simulink model "EV_Model"  (R2020b)
settings: Solver=VariableStepAuto  StartTime=0.0  StopTime=inf  RelTol=1e-3
undefined symbols (not defined in the file): battery, DCDC, DCU, DCU1, DiscIntNeverNeededParam, ECP, HVH, magnitude, PAR, PTC, road, SampleTime, VCU, veh, wheel
libraries: simulink x10
(part 1 of 2)
settings Model: SimulationMode=accelerator  Creator=LIKAI  LastModifiedBy=LIKAI

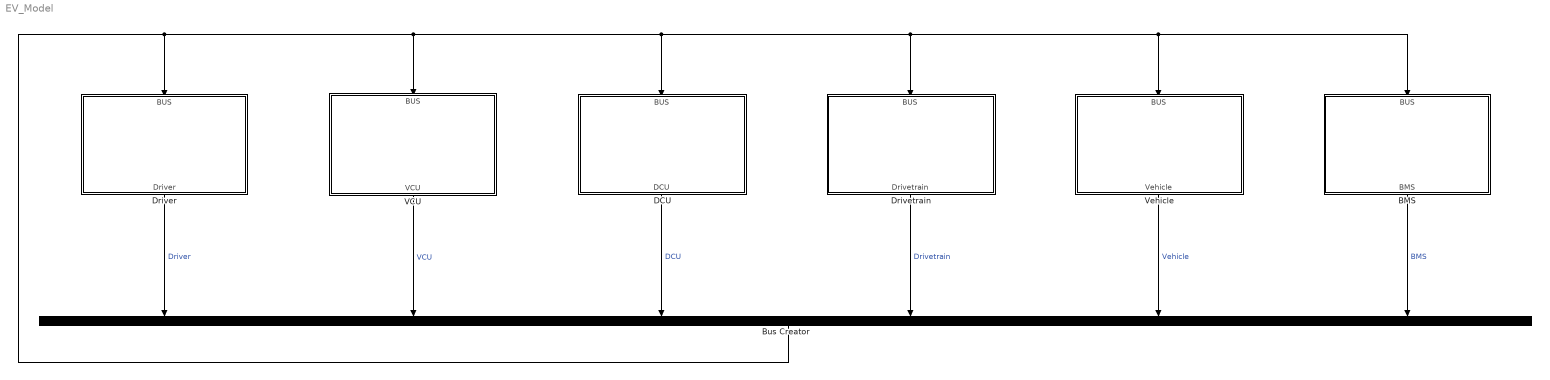
== system EV_Model ==
  BMS : Subsystem
      settings: PortSchema="{\"entries\":[{\"content\":{\"sides\":[{\"content\":{\"connectorIds\":[]},\"type\":\"ConnectorPlacement.EquallySpacedRectSide\",\"uuid\":\"ede90b11-bc22-42fb-ada4-d3cc8cd7e01b\"},{\"content\":{\"connectorIds\":[],\"side\":\"RIGHT\"},\"type\":\"ConnectorPlacement.EquallySpacedRectSide\",\"uuid\":\"291a790d-3ed9-499e-8b51-4c4b7bb0ca71\"},{\"content\":{\"connectorIds\":[\"In1\"],\"side\":\"TOP\"},\"type\":\"ConnectorPlacement.EquallySpacedRectSide\",\"uuid\":\"427db5b2-2806-4b1c-ab96-e85c737f1799\"},{\"content\":{\"connectorIds\":[\"Out1\"],\"side\":\"BOTTOM\"},\"type\":\"ConnectorPlacement.EquallySpacedRectSide\",\"uuid\":\"1165d243-ed6a-4f50-80fe-e5443602b1fc\"},{\"content\":{\"connectorIds\":[],\"side\":\"HIDDEN\"},\"type\":\"ConnectorPlacement.EquallySpacedRectSide\",\"uuid\":\"de95d8f7-8967-4dbd-bf20-0c2997ce61ce\"}]},\"type\":\"ConnectorPlacement.EquallySpacedConnector\",\"uuid\":\"60485ffc-06b9-4405-b269-3de14a5dc818\"}],\"packageUris\":[\"http://schema.mathworks.com/mf0/Connector/R2020b\"],\"version\":\"1.0\"}"
  Bus Creator : BusCreator  Inputs=6
  DCU : Subsystem
      settings: PortSchema="{\"entries\":[{\"content\":{\"sides\":[{\"content\":{\"connectorIds\":[]},\"type\":\"ConnectorPlacement.EquallySpacedRectSide\",\"uuid\":\"ede90b11-bc22-42fb-ada4-d3cc8cd7e01b\"},{\"content\":{\"connectorIds\":[],\"side\":\"RIGHT\"},\"type\":\"ConnectorPlacement.EquallySpacedRectSide\",\"uuid\":\"291a790d-3ed9-499e-8b51-4c4b7bb0ca71\"},{\"content\":{\"connectorIds\":[\"In1\"],\"side\":\"TOP\"},\"type\":\"ConnectorPlacement.EquallySpacedRectSide\",\"uuid\":\"427db5b2-2806-4b1c-ab96-e85c737f1799\"},{\"content\":{\"connectorIds\":[\"Out1\"],\"side\":\"BOTTOM\"},\"type\":\"ConnectorPlacement.EquallySpacedRectSide\",\"uuid\":\"f52060db-3c77-45a1-a434-e300d9b83897\"},{\"content\":{\"connectorIds\":[],\"side\":\"HIDDEN\"},\"type\":\"ConnectorPlacement.EquallySpacedRectSide\",\"uuid\":\"de95d8f7-8967-4dbd-bf20-0c2997ce61ce\"}]},\"type\":\"ConnectorPlacement.EquallySpacedConnector\",\"uuid\":\"60485ffc-06b9-4405-b269-3de14a5dc818\"}],\"packageUris\":[\"http://schema.mathworks.com/mf0/Connector/R2020b\"],\"version\":\"1.0\"}"
  Driver : Subsystem
      settings: PortSchema="{\"entries\":[{\"content\":{\"sides\":[{\"content\":{\"connectorIds\":[]},\"type\":\"ConnectorPlacement.EquallySpacedRectSide\",\"uuid\":\"ede90b11-bc22-42fb-ada4-d3cc8cd7e01b\"},{\"content\":{\"connectorIds\":[],\"side\":\"RIGHT\"},\"type\":\"ConnectorPlacement.EquallySpacedRectSide\",\"uuid\":\"291a790d-3ed9-499e-8b51-4c4b7bb0ca71\"},{\"content\":{\"connectorIds\":[\"In1\"],\"side\":\"TOP\"},\"type\":\"ConnectorPlacement.EquallySpacedRectSide\",\"uuid\":\"427db5b2-2806-4b1c-ab96-e85c737f1799\"},{\"content\":{\"connectorIds\":[\"Out1\"],\"side\":\"BOTTOM\"},\"type\":\"ConnectorPlacement.EquallySpacedRectSide\",\"uuid\":\"a05f4215-27ad-4dfe-901f-55fb3061c621\"},{\"content\":{\"connectorIds\":[],\"side\":\"HIDDEN\"},\"type\":\"ConnectorPlacement.EquallySpacedRectSide\",\"uuid\":\"de95d8f7-8967-4dbd-bf20-0c2997ce61ce\"}]},\"type\":\"ConnectorPlacement.EquallySpacedConnector\",\"uuid\":\"60485ffc-06b9-4405-b269-3de14a5dc818\"}],\"packageUris\":[\"http://schema.mathworks.com/mf0/Connector/R2020b\"],\"version\":\"1.0\"}"
  Drivetrain : Subsystem
      settings: PortSchema="{\"entries\":[{\"content\":{\"sides\":[{\"content\":{\"connectorIds\":[]},\"type\":\"ConnectorPlacement.EquallySpacedRectSide\",\"uuid\":\"ede90b11-bc22-42fb-ada4-d3cc8cd7e01b\"},{\"content\":{\"connectorIds\":[],\"side\":\"RIGHT\"},\"type\":\"ConnectorPlacement.EquallySpacedRectSide\",\"uuid\":\"291a790d-3ed9-499e-8b51-4c4b7bb0ca71\"},{\"content\":{\"connectorIds\":[\"In1\"],\"side\":\"TOP\"},\"type\":\"ConnectorPlacement.EquallySpacedRectSide\",\"uuid\":\"427db5b2-2806-4b1c-ab96-e85c737f1799\"},{\"content\":{\"connectorIds\":[\"Out1\"],\"side\":\"BOTTOM\"},\"type\":\"ConnectorPlacement.EquallySpacedRectSide\",\"uuid\":\"40f490df-ef26-4730-ad02-e07a11bb8b70\"},{\"content\":{\"connectorIds\":[],\"side\":\"HIDDEN\"},\"type\":\"ConnectorPlacement.EquallySpacedRectSide\",\"uuid\":\"de95d8f7-8967-4dbd-bf20-0c2997ce61ce\"}]},\"type\":\"ConnectorPlacement.EquallySpacedConnector\",\"uuid\":\"60485ffc-06b9-4405-b269-3de14a5dc818\"}],\"packageUris\":[\"http://schema.mathworks.com/mf0/Connector/R2020b\"],\"version\":\"1.0\"}"
  VCU : Subsystem
      settings: PortSchema="{\"entries\":[{\"content\":{\"sides\":[{\"content\":{\"connectorIds\":[]},\"type\":\"ConnectorPlacement.EquallySpacedRectSide\",\"uuid\":\"ede90b11-bc22-42fb-ada4-d3cc8cd7e01b\"},{\"content\":{\"connectorIds\":[],\"side\":\"RIGHT\"},\"type\":\"ConnectorPlacement.EquallySpacedRectSide\",\"uuid\":\"291a790d-3ed9-499e-8b51-4c4b7bb0ca71\"},{\"content\":{\"connectorIds\":[\"In1\"],\"side\":\"TOP\"},\"type\":\"ConnectorPlacement.EquallySpacedRectSide\",\"uuid\":\"427db5b2-2806-4b1c-ab96-e85c737f1799\"},{\"content\":{\"connectorIds\":[\"Out1\"],\"side\":\"BOTTOM\"},\"type\":\"ConnectorPlacement.EquallySpacedRectSide\",\"uuid\":\"15192dcd-7739-45f8-9f11-3c35b4b9a8fd\"},{\"content\":{\"connectorIds\":[],\"side\":\"HIDDEN\"},\"type\":\"ConnectorPlacement.EquallySpacedRectSide\",\"uuid\":\"de95d8f7-8967-4dbd-bf20-0c2997ce61ce\"}]},\"type\":\"ConnectorPlacement.EquallySpacedConnector\",\"uuid\":\"60485ffc-06b9-4405-b269-3de14a5dc818\"}],\"packageUris\":[\"http://schema.mathworks.com/mf0/Connector/R2020b\"],\"version\":\"1.0\"}"
  Vehicle : Subsystem
      settings: PortSchema="{\"entries\":[{\"content\":{\"sides\":[{\"content\":{\"connectorIds\":[]},\"type\":\"ConnectorPlacement.EquallySpacedRectSide\",\"uuid\":\"ede90b11-bc22-42fb-ada4-d3cc8cd7e01b\"},{\"content\":{\"connectorIds\":[],\"side\":\"RIGHT\"},\"type\":\"ConnectorPlacement.EquallySpacedRectSide\",\"uuid\":\"291a790d-3ed9-499e-8b51-4c4b7bb0ca71\"},{\"content\":{\"connectorIds\":[\"In1\"],\"side\":\"TOP\"},\"type\":\"ConnectorPlacement.EquallySpacedRectSide\",\"uuid\":\"427db5b2-2806-4b1c-ab96-e85c737f1799\"},{\"content\":{\"connectorIds\":[\"Out1\"],\"side\":\"BOTTOM\"},\"type\":\"ConnectorPlacement.EquallySpacedRectSide\",\"uuid\":\"01d5a7f7-95dc-4d6a-a6a5-fe54827ab0e5\"},{\"content\":{\"connectorIds\":[],\"side\":\"HIDDEN\"},\"type\":\"ConnectorPlacement.EquallySpacedRectSide\",\"uuid\":\"de95d8f7-8967-4dbd-bf20-0c2997ce61ce\"}]},\"type\":\"ConnectorPlacement.EquallySpacedConnector\",\"uuid\":\"60485ffc-06b9-4405-b269-3de14a5dc818\"}],\"packageUris\":[\"http://schema.mathworks.com/mf0/Connector/R2020b\"],\"version\":\"1.0\"}"
  wires:
  VCU/1(VCU) -> Bus Creator/2  "VCU"
  Driver/1(Driver) -> Bus Creator/1  "Driver"
  DCU/1(DCU) -> Bus Creator/3  "DCU"
  Drivetrain/1(Drivetrain) -> Bus Creator/4  "Drivetrain"
  Vehicle/1(Vehicle) -> Bus Creator/5  "Vehicle"
  BMS/1(BMS) -> Bus Creator/6  "BMS"
  Bus Creator/1 -> Drivetrain/1(BUS), BMS/1(BUS), Vehicle/1(BUS), DCU/1(BUS), VCU/1(BUS), Driver/1(BUS)

== system EV_Model/BMS ==
  BUS : Inport
  Battery Management System : Subsystem
  Bus Creator1 : BusCreator  Inputs=4
  Bus Selector : BusSelector  OutputSignals=Vehicle.AcesPwr_kW,Drivetrain.BattPwrReq_kW
  BMS : Outport  VectorParamsAs1DForOutWhenUnconnected=off
  wires:
  BUS/1 -> Bus Selector/1
  Battery Management System/1(BattSOC_1) -> Bus Creator1/1  "BattSOC_1"
  Battery Management System/2(BattVolt_V) -> Bus Creator1/2  "BattVolt_V"
  Battery Management System/3(BattPwrDischrgLmt_kW) -> Bus Creator1/3  "BattPwrDischrgLmt_kW"
  Battery Management System/4(BattPwrChrgLmt_kW) -> Bus Creator1/4  "BattPwrChrgLmt_kW"
  Bus Creator1/1 -> BMS/1
  Bus Selector/1 -> Battery Management System/1(AcesPwr_kW)  "<AcesPwr_kW>"
  Bus Selector/2 -> Battery Management System/2(BattPwrReq_kW)  "<BattPwrReq_kW>"

== system EV_Model/DCU ==
  BUS : Inport
  Bus Creator : BusCreator  Inputs=4
  Bus Selector : BusSelector  OutputSignals=BMS.BattVolt_V,Drivetrain.MotSpdAct_rpm,VCU.MotTrqReqBattPwrLimit_Nm
  Subsystem : Subsystem
  DCU : Outport  VectorParamsAs1DForOutWhenUnconnected=off
  wires:
  BUS/1 -> Bus Selector/1
  Bus Creator/1 -> DCU/1
  Subsystem/1(DCUTrqLimit_Nm) -> Bus Creator/1  "DCUTrqLimit_Nm"
  Subsystem/2(DCUPwrLimit_Nm) -> Bus Creator/2  "DCUPwrLimit_Nm"
  Subsystem/3(MotEffi2K_1) -> Bus Creator/3  "MotEffi2K_1"
  Subsystem/4(MotPwrElecReq_kW) -> Bus Creator/4  "MotPwrElecReq_kW"
  Bus Selector/1 -> Subsystem/1(BattVolt_V)  "<BattVolt_V>"
  Bus Selector/2 -> Subsystem/2(MotSpdAct_rpm)  "<MotSpdAct_rpm>"
  Bus Selector/3 -> Subsystem/3(MotTrqCmd_Nm)  "<MotTrqReqBattPwrLimit_Nm>"

== system EV_Model/Driver ==
  BUS : Inport
  Bus Creator : BusCreator  Inputs=2
  Bus Selector : BusSelector  OutputSignals=Vehicle.VehVelAct_kph
  DataTypeConversion1 : DataTypeConversion  OutDataTypeStr=double
  DataTypeConversion2 : DataTypeConversion  OutDataTypeStr=double
  DataTypeConversion6 : DataTypeConversion  OutDataTypeStr=double
  DriverModel : Subsystem
  Driver : Outport  VectorParamsAs1DForOutWhenUnconnected=off
  wires:
  Bus Selector/1 -> DataTypeConversion2/1  "<VehVelAct_kph>"
  DataTypeConversion2/1 -> DriverModel/1(VehVelAct_kph)
  DataTypeConversion1/1 -> Bus Creator/2  "WhlTrqCmd_Nm"
  DriverModel/1(VehVelTrgt_kph) -> DataTypeConversion6/1
  Bus Creator/1 -> Driver/1
  DriverModel/2(WhlTrqCmd_Nm) -> DataTypeConversion1/1
  BUS/1 -> Bus Selector/1
  DataTypeConversion6/1 -> Bus Creator/1  "VehVelTrgt_kph"

== system EV_Model/Drivetrain ==
  BUS : Inport
  Bus Creator : BusCreator  Inputs=4
  Bus Selector : BusSelector  OutputSignals=BMS.BattVolt_V,VCU.MotTrqFinalCmd_Nm,Vehicle.VehVelAct_kph
  Subsystem : Subsystem
  Drivetrain : Outport  VectorParamsAs1DForOutWhenUnconnected=off
  wires:
  Bus Creator/1 -> Drivetrain/1
  BUS/1 -> Bus Selector/1
  Subsystem/2(BattPwrReq_kW) -> Bus Creator/2  "BattPwrReq_kW"
  Subsystem/1(MotEffi_1) -> Bus Creator/1  "MotEffi_1"
  Subsystem/3(WheelTrqFromMot_Nm) -> Bus Creator/3  "WheelTrqFromMot_Nm"
  Subsystem/4(MotSpdAct_rpm) -> Bus Creator/4  "MotSpdAct_rpm"
  Bus Selector/3 -> Subsystem/3(VehVelAct_kph)  "<VehVelAct_kph>"
  Bus Selector/2 -> Subsystem/2(MotTrqCmd_Nm)  "<MotTrqFinalCmd_Nm>"
  Bus Selector/1 -> Subsystem/1(BattVolt_V)  "<BattVolt_V>"

== system EV_Model/VCU ==
  BUS : Inport
  Bus Creator : BusCreator  Inputs=2
  Bus Selector : BusSelector  OutputSignals=Driver.WhlTrqCmd_Nm,DCU.DCUTrqLimit_Nm,Vehicle.VehVelAct_kph,Drivetrain.MotSpdAct_rpm,DCU.MotPwrElecReq_kW,BMS.BattSOC_1,BMS.BattPwrDischrgLmt_kW,BMS.BattPwrChrgLmt_kW,DCU.MotEffi2K_1,DCU.DCUPwrLimit_Nm
  Subsystem : Subsystem
  VCU : Outport  VectorParamsAs1DForOutWhenUnconnected=off
  wires:
  BUS/1 -> Bus Selector/1
  Bus Creator/1 -> VCU/1
  Subsystem/1(MotTrqFinalCmd_Nm) -> Bus Creator/1  "MotTrqReqBattPwrLimit_Nm"
  Subsystem/2(MotTrqReqBattPwrLimit_Nm) -> Bus Creator/2  "MotTrqFinalCmd_Nm"
  Bus Selector/1 -> Subsystem/1(WhlTrqCmd_Nm)  "<WhlTrqCmd_Nm>"
  Bus Selector/4 -> Subsystem/4(MotSpdAct_rpm)  "<MotSpdAct_rpm>"
  Bus Selector/5 -> Subsystem/5(MotPwrElecReq_kW)  "<MotPwrElecReq_kW>"
  Bus Selector/6 -> Subsystem/6(BattSOC_1)  "<BattSOC_1>"
  Bus Selector/7 -> Subsystem/7(BattPwrDischrgLmt_kW)  "<BattPwrDischrgLmt_kW>"
  Bus Selector/8 -> Subsystem/8(BattPwrChrgLmt_kW)  "<BattPwrChrgLmt_kW>"
  Bus Selector/9 -> Subsystem/9(MotEffi2K_1)  "<MotEffi2K_1>"
  Bus Selector/10 -> Subsystem/10(DCUPwrLimit_Nm)  "<DCUPwrLimit_Nm>"
  Bus Selector/2 -> Subsystem/2(DCUTrqLimit_Nm)  "<DCUTrqLimit_Nm>"
  Bus Selector/3 -> Subsystem/3(VehVelAct_kph)  "<VehVelAct_kph>"

== system EV_Model/Vehicle ==
  BUS : Inport
  Bus Creator : BusCreator  Inputs=5
  Bus Selector : BusSelector  OutputSignals=Drivetrain.WheelTrqFromMot_Nm,Driver.WhlTrqCmd_Nm
  DCDC : Subsystem
  Dynamic : Subsystem
  Vehicle : Outport  VectorParamsAs1DForOutWhenUnconnected=off
  wires:
  Bus Creator/1 -> Vehicle/1
  BUS/1 -> Bus Selector/1
  Dynamic/1(VehVelAct_kph) -> Bus Creator/2  "VehVelAct_kph"
  Dynamic/2(VehAccAct_m/s^2) -> Bus Creator/3  "VehAccAct_m/s^2"
  Dynamic/3(FricBrakeTrq_Nm) -> Bus Creator/4  "FricBrakeTrq_Nm"
  Dynamic/4(WheelTrqAct_Nm) -> Bus Creator/5  "WheelTrqAct_Nm"
  DCDC/1(AcesPwr_kW) -> Bus Creator/1  "AcesPwr_kW"
  Bus Selector/1 -> Dynamic/1(WheelTrqFromMot_Nm)  "<WheelTrqFromMot_Nm>"
  Bus Selector/2 -> Dynamic/2(WhlTrqCmd_Nm)  "<WhlTrqCmd_Nm>"

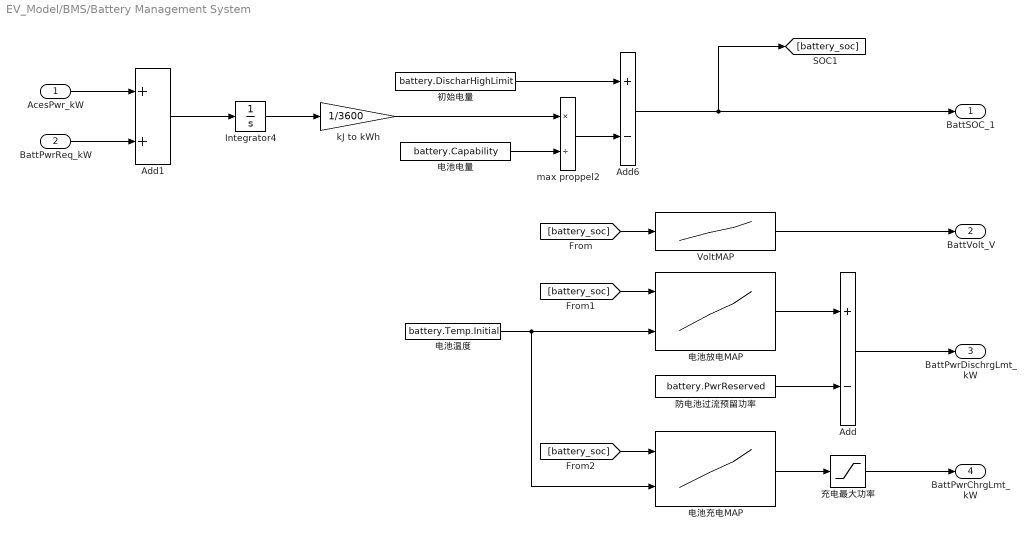
== system EV_Model/BMS/Battery Management System ==
  AcesPwr_kW : Inport
  BattPwrReq_kW : Inport  Port=2
  Add : Sum  Inputs=+-
  Add1 : Sum
  Add6 : Sum  Inputs=+-
  Integrator4 : Integrator
  VoltMAP : Lookup_n-D  NumberOfTableDimensions=1  BreakpointsForDimension1=battery.VoltMap.SOC  BreakpointsForDimension2=DCU.EffMap.map1.SpdTab  Table=battery.VoltMap.Volt  InternalRulePriority=Speed  RndMeth=Simplest  InputSameDT=on
  kJ to kWh : Gain  Gain=1/3600
  max proppel2 : Product  Inputs=*/
  充电最大功率 : Saturate  UpperLimit=150  LowerLimit=0
  初始电量 : Constant  Value=battery.DischarHighLimit
  电池充电MAP : Lookup_n-D  BreakpointsForDimension1=battery.ChaPwrMap.SOC  BreakpointsForDimension2=battery.ChaPwrMap.Temp  Table=battery.ChaPwrMap.Pwr  InternalRulePriority=Speed  RndMeth=Simplest  InputSameDT=on
      settings: InputPortMap=u0,u1
  电池放电MAP : Lookup_n-D  BreakpointsForDimension1=battery.DischaPwrMap.SOC  BreakpointsForDimension2=battery.DischaPwrMap.Temp  Table=battery.DischaPwrMap.Pwr  InternalRulePriority=Speed  RndMeth=Simplest  InputSameDT=on
      settings: InputPortMap=u0,u1
  电池温度 : Constant  Value=battery.Temp.Initial
  电池电量 : Constant  Value=battery.Capability
  防电池过流预留功率 : Constant  Value=battery.PwrReserved
  BattSOC_1 : Outport
  BattVolt_V : Outport  Port=2
  BattPwrDischrgLmt_kW : Outport  Port=3  VectorParamsAs1DForOutWhenUnconnected=off
  BattPwrChrgLmt_kW : Outport  Port=4  VectorParamsAs1DForOutWhenUnconnected=off
  wires:
  防电池过流预留功率/1 -> Add/2
  电池放电MAP/1 -> Add/1
  电池温度/1 -> 电池充电MAP/2, 电池放电MAP/2
  电池充电MAP/1 -> 充电最大功率/1
  VoltMAP/1 -> BattVolt_V/1
  初始电量/1 -> Add6/1
  电池电量/1 -> max proppel2/2
  max proppel2/1 -> Add6/2
  Add6/1 -> BattSOC_1/1, [battery_soc]
  [battery_soc] -> VoltMAP/1
  [battery_soc] -> 电池放电MAP/1
  [battery_soc] -> 电池充电MAP/1
  Add/1 -> BattPwrDischrgLmt_kW/1
  充电最大功率/1 -> BattPwrChrgLmt_kW/1
  AcesPwr_kW/1 -> Add1/1
  BattPwrReq_kW/1 -> Add1/2
  Add1/1 -> Integrator4/1
  Integrator4/1 -> kJ to kWh/1
  kJ to kWh/1 -> max proppel2/1

== system EV_Model/DCU/Subsystem ==
  BattVolt_V : Inport
  MotSpdAct_rpm : Inport  Port=2
  MotTrqCmd_Nm : Inport  Port=3
  DCUPwrLimit : Subsystem
  DCUPwrReq : Subsystem
  DCUTrqLimit : Subsystem
  DCUTrqLimit_Nm : Outport
  DCUPwrLimit_Nm : Outport  Port=2
  MotEffi2K_1 : Outport  Port=3
  MotPwrElecReq_kW : Outport  Port=4
  wires:
  MotTrqCmd_Nm/1 -> DCUPwrReq/3(MotTrqCmd_Nm)
  BattVolt_V/1 -> DCUPwrReq/1(BattVolt_V), DCUPwrLimit/1(BattVolt_V), DCUTrqLimit/1(BattVolt_V)
  DCUPwrReq/1(MotEffi2K_1) -> MotEffi2K_1/1
  DCUPwrLimit/1(DCUPwrLimit_Nm) -> DCUPwrLimit_Nm/1
  MotSpdAct_rpm/1 -> DCUPwrReq/2(MotSpdAct_rpm), DCUPwrLimit/2(MotSpdAct_rpm), DCUTrqLimit/2(MotSpdAct_rpm)
  DCUPwrReq/2(MotPwrElecReq_kW) -> MotPwrElecReq_kW/1
  DCUTrqLimit/1(DCUTrqLimit_Nm) -> DCUTrqLimit_Nm/1

== system EV_Model/Driver/DriverModel ==
  VehVelAct_kph : Inport
  PID : Subsystem
  Sum5 : Sum
  WhlTrqCal : Subsystem
  VehVelTrgt_kph : Outport  VectorParamsAs1DForOutWhenUnconnected=off
  WhlTrqCmd_Nm : Outport  Port=2  VectorParamsAs1DForOutWhenUnconnected=off
  wires:
  WhlTrqCal/1(VehVelTrgt_kph) -> VehVelTrgt_kph/1, PID/1(VehVelTrgt_kph)
  VehVelAct_kph/1 -> PID/2(VehVelAct_kph)
  PID/1(PIDTrq_Nm) -> Sum5/1
  WhlTrqCal/2(WhlTrqReq_Nm) -> Sum5/2
  Sum5/1 -> WhlTrqCmd_Nm/1  "PI控制后的轮端扭矩需求"

== system EV_Model/Drivetrain/Subsystem ==
  BattVolt_V : Inport
  MotTrqCmd_Nm : Inport  Port=2
  VehVelAct_kph : Inport  Port=3
  Final Drive : Subsystem
  MOTOR : Subsystem
  Speed Calculation : Subsystem
  MotEffi_1 : Outport
  BattPwrReq_kW : Outport  Port=2
  WheelTrqFromMot_Nm : Outport  Port=3
  MotSpdAct_rpm : Outport  Port=4
  wires:
  MOTOR/3(MotTrqAct_Nm) -> Final Drive/1(MotTrqAct_Nm)
  MotTrqCmd_Nm/1 -> MOTOR/2(MotTrqCmd_Nm)
  MOTOR/1(MotEffi_1) -> MotEffi_1/1
  Speed Calculation/1(MotSpdAct_rpm) -> MotSpdAct_rpm/1, MOTOR/3(MotSpdAct_rpm)
  BattVolt_V/1 -> MOTOR/1(BattVolt_V)
  Final Drive/1(WheelTrqFromMot_Nm) -> WheelTrqFromMot_Nm/1
  MOTOR/2(BattPwrReq_kW) -> BattPwrReq_kW/1
  VehVelAct_kph/1 -> Speed Calculation/1(VehVelAct_kph)

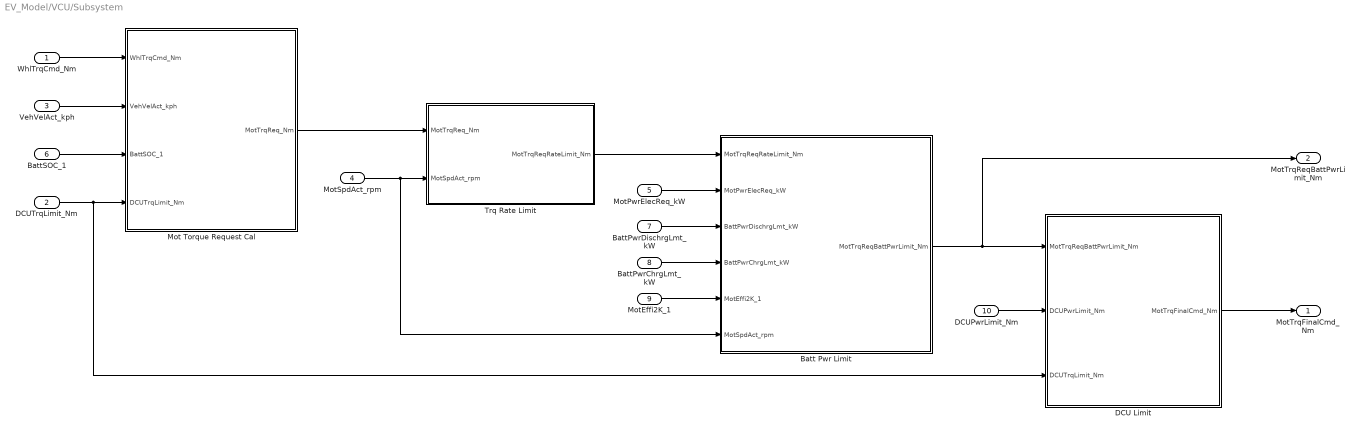
== system EV_Model/VCU/Subsystem ==
  WhlTrqCmd_Nm : Inport
  DCUTrqLimit_Nm : Inport  Port=2
  VehVelAct_kph : Inport  Port=3
  MotSpdAct_rpm : Inport  Port=4
  MotPwrElecReq_kW : Inport  Port=5
  BattSOC_1 : Inport  Port=6
  BattPwrDischrgLmt_kW : Inport  Port=7
  BattPwrChrgLmt_kW : Inport  Port=8
  MotEffi2K_1 : Inport  Port=9
  DCUPwrLimit_Nm : Inport  Port=10
  Batt Pwr Limit : Subsystem
  DCU Limit : Subsystem
  Mot Torque Request Cal : Subsystem
  Trq Rate Limit : Subsystem
  MotTrqFinalCmd_Nm : Outport
  MotTrqReqBattPwrLimit_Nm : Outport  Port=2
  wires:
  Batt Pwr Limit/1(MotTrqReqBattPwrLimit_Nm) -> MotTrqReqBattPwrLimit_Nm/1, DCU Limit/1(MotTrqReqBattPwrLimit_Nm)
  BattPwrChrgLmt_kW/1 -> Batt Pwr Limit/4(BattPwrChrgLmt_kW)
  Trq Rate Limit/1(MotTrqReqRateLimit_Nm) -> Batt Pwr Limit/1(MotTrqReqRateLimit_Nm)
  Mot Torque Request Cal/1(MotTrqReq_Nm) -> Trq Rate Limit/1(MotTrqReq_Nm)
  MotSpdAct_rpm/1 -> Trq Rate Limit/2(MotSpdAct_rpm), Batt Pwr Limit/6(MotSpdAct_rpm)
  MotPwrElecReq_kW/1 -> Batt Pwr Limit/2(MotPwrElecReq_kW)
  DCU Limit/1(MotTrqFinalCmd_Nm) -> MotTrqFinalCmd_Nm/1
  DCUPwrLimit_Nm/1 -> DCU Limit/2(DCUPwrLimit_Nm)
  DCUTrqLimit_Nm/1 -> DCU Limit/3(DCUTrqLimit_Nm), Mot Torque Request Cal/4(DCUTrqLimit_Nm)
  BattSOC_1/1 -> Mot Torque Request Cal/3(BattSOC_1)
  BattPwrDischrgLmt_kW/1 -> Batt Pwr Limit/3(BattPwrDischrgLmt_kW)
  MotEffi2K_1/1 -> Batt Pwr Limit/5(MotEffi2K_1)
  WhlTrqCmd_Nm/1 -> Mot Torque Request Cal/1(WhlTrqCmd_Nm)
  VehVelAct_kph/1 -> Mot Torque Request Cal/2(VehVelAct_kph)

== system EV_Model/Vehicle/DCDC ==
  Add1 : Sum  Inputs=++++
  DC-DC efficiency : Constant  Value=DCDC.Eff
  W to kW : Gain  Gain=1000
  max proppel1 : Product  Inputs=*/
  低压负载 : Constant  Value=veh.LvPwr
  热敏电阻加热 : Constant  Value=PTC.Pwr
  电动水泵 : Constant  Value=ECP.Pwr
  高压电池加热 : Constant  Value=HVH.Pwr
  AcesPwr_kW : Outport
  wires:
  max proppel1/1 -> Add1/1
  DC-DC efficiency/1 -> max proppel1/2
  热敏电阻加热/1 -> Add1/2
  低压负载/1 -> max proppel1/1
  高压电池加热/1 -> Add1/3
  电动水泵/1 -> Add1/4
  Add1/1 -> W to kW/1
  W to kW/1 -> AcesPwr_kW/1

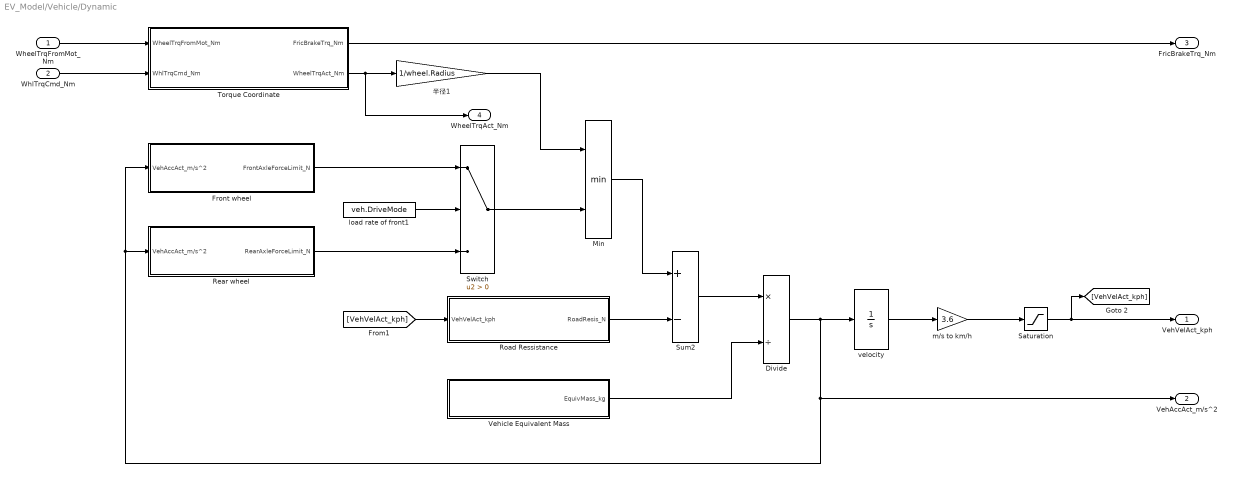
== system EV_Model/Vehicle/Dynamic ==
  WheelTrqFromMot_Nm : Inport
  WhlTrqCmd_Nm : Inport  Port=2
  Divide : Product  Inputs=*/
  Front wheel : Subsystem
  Min : MinMax  Inputs=2
  Rear wheel : Subsystem
  Road Ressistance : Subsystem
  Saturation : Saturate  UpperLimit=inf  LowerLimit=0
  Sum2 : Sum  Inputs=+-
  Switch : Switch  Criteria=u2 > Threshold
  Torque Coordinate : Subsystem
  Vehicle Equivalent Mass : Subsystem
  load rate of front1 : Constant  Value=veh.DriveMode
  m/s to km/h : Gain  Gain=3.6
  velocity : Integrator
  半径1 : Gain  Gain=1/wheel.Radius
  VehVelAct_kph : Outport
  VehAccAct_m/s^2 : Outport  Port=2
  FricBrakeTrq_Nm : Outport  Port=3
  WheelTrqAct_Nm : Outport  Port=4
  wires:
  Front wheel/1(FrontAxleForceLimit_N) -> Switch/1
  Rear wheel/1(RearAxleForceLimit_N) -> Switch/3
  load rate of front1/1 -> Switch/2
  WheelTrqFromMot_Nm/1 -> Torque Coordinate/1(WheelTrqFromMot_Nm)
  WhlTrqCmd_Nm/1 -> Torque Coordinate/2(WhlTrqCmd_Nm)
  Switch/1 -> Min/2
  Torque Coordinate/2(WheelTrqAct_Nm) -> WheelTrqAct_Nm/1, 半径1/1
  半径1/1 -> Min/1
  Road Ressistance/1(RoadResis_N) -> Sum2/2
  Min/1 -> Sum2/1
  Sum2/1 -> Divide/1
  Vehicle Equivalent Mass/1(EquivMass_kg) -> Divide/2
  Divide/1 -> VehAccAct_m/s^2/1, Front wheel/1(VehAccAct_m/s^2), Rear wheel/1(VehAccAct_m/s^2), velocity/1
  velocity/1 -> m/s to km/h/1
  m/s to km/h/1 -> Saturation/1
  Saturation/1 -> [VehVelAct_kph], VehVelAct_kph/1
  [VehVelAct_kph] -> Road Ressistance/1(VehVelAct_kph)
  Torque Coordinate/1(FricBrakeTrq_Nm) -> FricBrakeTrq_Nm/1

== system EV_Model/DCU/Subsystem/DCUPwrLimit ==
  BattVolt_V : Inport
  MotSpdAct_rpm : Inport  Port=2
  "Crossfade " : Subsystem  AncestorBlock=GAC_library/Crossfade  mask(Crossfade){}
      mask help: Gradual changing of output in accordance with input siganl F. When the input signal F equals MX, Out equals max. When the input signal F equals NRM, Out equals norm. When the input signal F equals MN, Out equals min. When signal F is between the nominated values of MX/NRM or MN/NRM, then output executes liner interpolation.
      mask Display:
      | color('black')
      | port_label('input', 1, 'F');
      | port_label('input', 2, 'max');
      | port_label('input', 3, 'norm');
      | port_label('input', 4, 'min');
      | port_label('input', 5, 'MX');
      | port_label('input', 6, 'NRM');
      | port_label('input', 7, 'MN');
      | port_label('output',1, 'out');
      | plot(100,100);
      | plot(0,0);
      | color('blue');
      | plot([40 70],[20 20]);
      | plot([40 70],[50 50]);
      | plot([40 70],[80 80]);
      | plot([55 55],[20 80]);
      | text(30,20,'-1');
      | text(30,50,'0');
      | text(30,80,'1');
  Divide : Product  Inputs=*/
  Gain : Gain  Gain=9549
  constant2 : Constant  Value=DCU1.EffMap.map1.Volt
  constant3 : Constant  Value=DCU1.EffMap.map2.Volt
  constant4 : Constant  Value=DCU1.EffMap.map3.Volt
  电驱外特性(Medium SOC) : Lookup_n-D  NumberOfTableDimensions=1  BreakpointsForDimension1=DCU1.TrqAbility.map2.spdTab  Table=DCU1.TrqAbility.map2.trqTab  InternalRulePriority=Speed  RndMeth=Simplest  InputSameDT=on
  电驱外特性(highSOC) : Lookup_n-D  NumberOfTableDimensions=1  BreakpointsForDimension1=DCU1.TrqAbility.map1.spdTab  Table=DCU1.TrqAbility.map1.trqTab  InternalRulePriority=Speed  RndMeth=Simplest  InputSameDT=on
  电驱外特性(low SOC) : Lookup_n-D  NumberOfTableDimensions=1  BreakpointsForDimension1=DCU1.TrqAbility.map3.spdTab  Table=DCU1.TrqAbility.map3.trqTab  InternalRulePriority=Speed  RndMeth=Simplest  InputSameDT=on
  DCUPwrLimit_Nm : Outport  VectorParamsAs1DForOutWhenUnconnected=off
  wires:
  constant3/1 -> "Crossfade "/6("norm_in ")
  constant2/1 -> "Crossfade "/5(max_in)
  constant4/1 -> "Crossfade "/7(min_in)
  电驱外特性(highSOC)/1 -> "Crossfade "/2(max_out)
  MotSpdAct_rpm/1 -> 电驱外特性(highSOC)/1, Divide/2, 电驱外特性(low SOC)/1, 电驱外特性(Medium SOC)/1
  BattVolt_V/1 -> "Crossfade "/1(F_in)
  电驱外特性(low SOC)/1 -> "Crossfade "/4(min_out)
  电驱外特性(Medium SOC)/1 -> "Crossfade "/3("norm_out ")
  "Crossfade "/1(Output) -> Gain/1
  Gain/1 -> Divide/1
  Divide/1 -> DCUPwrLimit_Nm/1

== system EV_Model/DCU/Subsystem/DCUPwrReq ==
  BattVolt_V : Inport
  MotSpdAct_rpm : Inport  Port=2
  MotTrqCmd_Nm : Inport  Port=3
  Efficiency : Subsystem
  Power : Subsystem
  MotEffi2K_1 : Outport  VectorParamsAs1DForOutWhenUnconnected=off
  MotPwrElecReq_kW : Outport  Port=2  VectorParamsAs1DForOutWhenUnconnected=off
  wires:
  MotTrqCmd_Nm/1 -> Power/3(MotTrqCmd_Nm), Efficiency/2(MotTrqCmd_Nm)
  BattVolt_V/1 -> Efficiency/1(BattVolt_V)
  MotSpdAct_rpm/1 -> Efficiency/3(MotSpdAct_rpm), Power/2(MotSpdAct_rpm)
  Efficiency/1(MotEffi_1) -> Power/1(MotEffi_1)
  Power/1(MotPwrElecReq_kW) -> MotPwrElecReq_kW/1
  Power/2(MotEffi2K_1) -> MotEffi2K_1/1

== system EV_Model/DCU/Subsystem/DCUTrqLimit ==
  BattVolt_V : Inport
  MotSpdAct_rpm : Inport  Port=2
  "Crossfade " : Subsystem  AncestorBlock=GAC_library/Crossfade  mask(Crossfade){}
      mask help: Gradual changing of output in accordance with input siganl F. When the input signal F equals MX, Out equals max. When the input signal F equals NRM, Out equals norm. When the input signal F equals MN, Out equals min. When signal F is between the nominated values of MX/NRM or MN/NRM, then output executes liner interpolation.
      mask Display:
      | color('black')
      | port_label('input', 1, 'F');
      | port_label('input', 2, 'max');
      | port_label('input', 3, 'norm');
      | port_label('input', 4, 'min');
      | port_label('input', 5, 'MX');
      | port_label('input', 6, 'NRM');
      | port_label('input', 7, 'MN');
      | port_label('output',1, 'out');
      | plot(100,100);
      | plot(0,0);
      | color('blue');
      | plot([40 70],[20 20]);
      | plot([40 70],[50 50]);
      | plot([40 70],[80 80]);
      | plot([55 55],[20 80]);
      | text(30,20,'-1');
      | text(30,50,'0');
      | text(30,80,'1');
  constant2 : Constant  Value=DCU1.EffMap.map1.Volt
  constant3 : Constant  Value=DCU1.EffMap.map2.Volt
  constant4 : Constant  Value=DCU1.EffMap.map3.Volt
  电驱外特性(Medium SOC) : Lookup_n-D  NumberOfTableDimensions=1  BreakpointsForDimension1=DCU1.TrqAbility.map2.spdTab  Table=DCU1.TrqAbility.map2.trqTab  InternalRulePriority=Speed  RndMeth=Simplest  InputSameDT=on
  电驱外特性(highSOC) : Lookup_n-D  NumberOfTableDimensions=1  BreakpointsForDimension1=DCU1.TrqAbility.map1.spdTab  Table=DCU1.TrqAbility.map1.trqTab  InternalRulePriority=Speed  RndMeth=Simplest  InputSameDT=on
  电驱外特性(low SOC) : Lookup_n-D  NumberOfTableDimensions=1  BreakpointsForDimension1=DCU1.TrqAbility.map3.spdTab  Table=DCU1.TrqAbility.map3.trqTab  InternalRulePriority=Speed  RndMeth=Simplest  InputSameDT=on
  DCUTrqLimit_Nm : Outport  VectorParamsAs1DForOutWhenUnconnected=off
  wires:
  电驱外特性(low SOC)/1 -> "Crossfade "/4(min_out)
  constant2/1 -> "Crossfade "/5(max_in)
  MotSpdAct_rpm/1 -> 电驱外特性(highSOC)/1, 电驱外特性(low SOC)/1, 电驱外特性(Medium SOC)/1
  电驱外特性(Medium SOC)/1 -> "Crossfade "/3("norm_out ")
  constant3/1 -> "Crossfade "/6("norm_in ")
  "Crossfade "/1(Output) -> DCUTrqLimit_Nm/1
  电驱外特性(highSOC)/1 -> "Crossfade "/2(max_out)
  BattVolt_V/1 -> "Crossfade "/1(F_in)
  constant4/1 -> "Crossfade "/7(min_in)

== system EV_Model/Driver/DriverModel/PID ==
  VehVelTrgt_kph : Inport
  VehVelAct_kph : Inport  Port=2
  1 : Product  InputSameDT=on  SaturateOnIntegerOverflow=on  OutDataTypeStr=Inherit: Same as first input
  Add2 : Sum  Inputs=+-
  Compare ToZero : simulink/Logic and Bit Operations/Compare To Zero  relop=>  OutDataTypeStr=boolean
  Compare ToZero1 : simulink/Logic and Bit Operations/Compare To Zero  relop=<=  OutDataTypeStr=boolean
  DataTypeConversion : DataTypeConversion  OutDataTypeStr=double
  Memory : Memory
  PIDACC : Subsystem  mask(PID Controller){P=200, I=20, D=0, initial=0, max=1, min=-1}
      mask prompts: P "Proportional:"; I "Integral:"; D "Derivative:"; initial "Initial value"; max "Range max value"; min "Range min value"
      mask help:
      | Enter expressions for proportional, integral, and derivative terms.
      | P+I/s+Ds
      mask Help: This block implements a PID controller where parameters are entered for the Proportional, Integral and Derivative terms. Unmask this block to see how it works. The derivative term is implemented using a true derivative block.
      mask Display:
      | % disp('PID')
      | color('blue');
      | fprintf('  PID  ');
      | color('red');
      | text(1,0,'GAC','horizontalAlignment','right','verticalAlignment','bottom');
  Product : Product
  PIDTrq_Nm : Outport  VectorParamsAs1DForOutWhenUnconnected=off
  wires:
  Compare ToZero1/1 -> PIDACC/2(reset)
  Add2/1 -> 1/2
  PIDACC/1(Out_1) -> PIDTrq_Nm/1
  1/1 -> Memory/1, Product/1, PIDACC/1(Error)
  Compare ToZero/1 -> DataTypeConversion/1
  DataTypeConversion/1 -> 1/1
  Memory/1 -> Product/2
  Product/1 -> Compare ToZero1/1
  VehVelAct_kph/1 -> Add2/2
  VehVelTrgt_kph/1 -> Compare ToZero/1, Add2/1

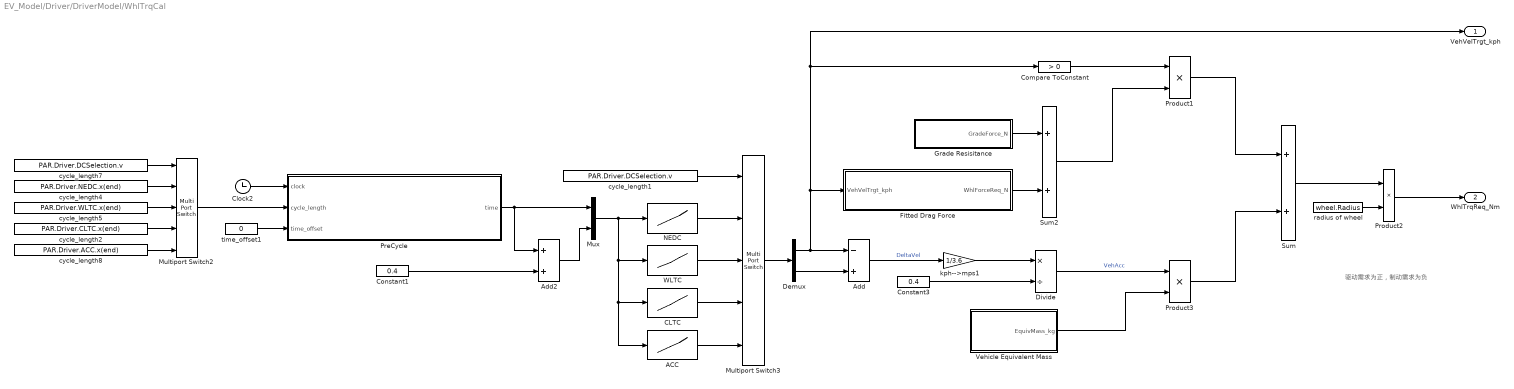
== system EV_Model/Driver/DriverModel/WhlTrqCal ==
  note: 驱动需求为正，制动需求为负
  ACC : Lookup  InputValues=PAR.Driver.ACC.x  Table=PAR.Driver.ACC.v  LookUpMeth=Interpolation-Use End Values
  Add : Sum  Inputs=-+
  Add2 : Sum
  CLTC : Lookup  InputValues=PAR.Driver.CLTC.x  Table=PAR.Driver.CLTC.v  LookUpMeth=Interpolation-Use End Values
  Clock2 : Clock
  Compare ToConstant : simulink/Logic and Bit Operations/Compare To Constant  relop=>  const=0  OutDataTypeStr=boolean
  Constant1 : Constant  Value=0.4  SampleTime=-1
  Constant3 : Constant  Value=0.4  SampleTime=-1
  Demux : Demux  Outputs=2
  Divide : Product  Inputs=*/
  "Fitted Drag Force " : Subsystem
  Grade Resisitance : Subsystem
  Multiport Switch2 : MultiPortSwitch  DataPortOrder=Zero-based contiguous  Inputs=4  zeroidx=on
  Multiport Switch3 : MultiPortSwitch  DataPortOrder=Zero-based contiguous  Inputs=4  zeroidx=on
  Mux : Mux  Inputs=2
  NEDC : Lookup  InputValues=PAR.Driver.NEDC.x  Table=PAR.Driver.NEDC.v  LookUpMeth=Interpolation-Use End Values
  PreCycle : Subsystem
  Product1 : Product
  Product2 : Product  Inputs=**
  Product3 : Product
  Sum : Sum
  Sum2 : Sum
  Vehicle Equivalent Mass : Subsystem
  WLTC : Lookup  InputValues=PAR.Driver.WLTC.x  Table=PAR.Driver.WLTC.v  LookUpMeth=Interpolation-Use End Values
  cycle_length1 : Constant  Value=PAR.Driver.DCSelection.v  SampleTime=-1
  cycle_length2 : Constant  Value=PAR.Driver.CLTC.x(end)  SampleTime=-1
  cycle_length4 : Constant  Value=PAR.Driver.NEDC.x(end)  SampleTime=-1
  cycle_length5 : Constant  Value=PAR.Driver.WLTC.x(end)  SampleTime=-1
  cycle_length7 : Constant  Value=PAR.Driver.DCSelection.v  SampleTime=-1
  cycle_length8 : Constant  Value=PAR.Driver.ACC.x(end)  SampleTime=-1
  kph-->mps1 : Gain  Gain=1/3.6
  radius of wheel : Constant  Value=wheel.Radius
  time_offset1 : Constant  Value=0  SampleTime=-1
  VehVelTrgt_kph : Outport  VectorParamsAs1DForOutWhenUnconnected=off
  WhlTrqReq_Nm : Outport  Port=2  VectorParamsAs1DForOutWhenUnconnected=off
  wires:
  Demux/2 -> Add/2
  PreCycle/1(time) -> Mux/1, Add2/1
  Add2/1 -> Mux/2
  Mux/1 -> ACC/1, CLTC/1, WLTC/1, NEDC/1
  Add/1 -> kph-->mps1/1  "DeltaVel"
  kph-->mps1/1 -> Divide/1
  Demux/1 -> Add/1, VehVelTrgt_kph/1, Compare ToConstant/1, "Fitted Drag Force "/1(VehVelTrgt_kph)
  time_offset1/1 -> PreCycle/3(time_offset)
  Clock2/1 -> PreCycle/1(clock)
  Multiport Switch2/1 -> PreCycle/2(cycle_length)
  Compare ToConstant/1 -> Product1/1
  Multiport Switch3/1 -> Demux/1
  Constant1/1 -> Add2/2
  Constant3/1 -> Divide/2
  cycle_length7/1 -> Multiport Switch2/1
  cycle_length5/1 -> Multiport Switch2/3
  cycle_length4/1 -> Multiport Switch2/2
  cycle_length1/1 -> Multiport Switch3/1
  NEDC/1 -> Multiport Switch3/2
  WLTC/1 -> Multiport Switch3/3
  cycle_length2/1 -> Multiport Switch2/4
  cycle_length8/1 -> Multiport Switch2/5
  CLTC/1 -> Multiport Switch3/4
  ACC/1 -> Multiport Switch3/5
  radius of wheel/1 -> Product2/2
  Product2/1 -> WhlTrqReq_Nm/1
  Grade Resisitance/1(GradeForce_N) -> Sum2/1
  "Fitted Drag Force "/1(WhlForceReq_N) -> Sum2/2
  Sum2/1 -> Product1/2
  Divide/1 -> Product3/1  "VehAcc"
  Vehicle Equivalent Mass/1(EquivMass_kg) -> Product3/2
  Product1/1 -> Sum/1
  Product3/1 -> Sum/2
  Sum/1 -> Product2/1

== system EV_Model/Drivetrain/Subsystem/Final Drive ==
  MotTrqAct_Nm : Inport
  Product1 : Product  Inputs=**
  Product2 : Product  Inputs=**
  Product3 : Product  Inputs=*/
  final drive : Constant  Value=DCU1.FdRatio
  finaldrive efficiency1 : Constant  Value=DCU1.FdEff
  finaldrive efficiency2 : Constant  Value=DCU1.FdEff
  驱动or回收 : Switch
  WheelTrqFromMot_Nm : Outport
  wires:
  Product3/1 -> 驱动or回收/3
  Product1/1 -> Product2/2, 驱动or回收/2, Product3/1
  final drive/1 -> Product1/2
  finaldrive efficiency1/1 -> Product3/2
  Product2/1 -> 驱动or回收/1
  驱动or回收/1 -> WheelTrqFromMot_Nm/1
  finaldrive efficiency2/1 -> Product2/1
  MotTrqAct_Nm/1 -> Product1/1

== system EV_Model/Drivetrain/Subsystem/MOTOR ==
  BattVolt_V : Inport
  MotTrqCmd_Nm : Inport  Port=2
  MotSpdAct_rpm : Inport  Port=3
  Efficiency : Subsystem
  MotTrqFilter : Subsystem
  Power : Subsystem
  MotEffi_1 : Outport  VectorParamsAs1DForOutWhenUnconnected=off
  BattPwrReq_kW : Outport  Port=2  VectorParamsAs1DForOutWhenUnconnected=off
  MotTrqAct_Nm : Outport  Port=3  VectorParamsAs1DForOutWhenUnconnected=off
  wires:
  MotTrqCmd_Nm/1 -> MotTrqFilter/1(MotTrqCmd_Nm), Power/3(MotTrqCmd_Nm), Efficiency/2(MotTrqCmd_Nm)
  BattVolt_V/1 -> Efficiency/1(BattVolt_V)
  MotSpdAct_rpm/1 -> Efficiency/3(MotSpdAct_rpm), Power/2(MotSpdAct_rpm)
  Efficiency/1(MotEffi_1) -> MotEffi_1/1, Power/1(MotEffi_1)
  Power/1(BattPwrReq_kW) -> BattPwrReq_kW/1
  MotTrqFilter/1(MotTrqCmdFilter_Nm) -> MotTrqAct_Nm/1

== system EV_Model/Drivetrain/Subsystem/Speed Calculation ==
  VehVelAct_kph : Inport
  final drive3 : Constant  Value=DCU1.FdRatio
  max proppel4 : Product  Inputs=*/*/
  radius of wheel3 : Constant  Value=wheel.Radius
  unit conversion factor3 : Constant  Value=0.377
  MotSpdAct_rpm : Outport
  wires:
  final drive3/1 -> max proppel4/3
  radius of wheel3/1 -> max proppel4/2
  unit conversion factor3/1 -> max proppel4/4
  max proppel4/1 -> MotSpdAct_rpm/1
  VehVelAct_kph/1 -> max proppel4/1

== system EV_Model/VCU/Subsystem/Batt Pwr Limit ==
  MotTrqReqRateLimit_Nm : Inport
  MotPwrElecReq_kW : Inport  Port=2
  BattPwrDischrgLmt_kW : Inport  Port=3
  BattPwrChrgLmt_kW : Inport  Port=4
  MotEffi2K_1 : Inport  Port=5
  MotSpdAct_rpm : Inport  Port=6
  Abs : Abs
  Check Within Limits : Subsystem
  Compare To Constant : simulink/Logic and Bit Operations/Compare To Constant  relop=<  const=2  OutDataTypeStr=boolean
  ElecToMechPwr : Product  Inputs=*/
  MechPwrToTrq : Product  Inputs=*/
  Switch : Switch  Criteria=u2 > Threshold
  Switch1 : Switch  Criteria=u2 > Threshold
  MotTrqReqBattPwrLimit_Nm : Outport
  wires:
  MotPwrElecReq_kW/1 -> Check Within Limits/2(u)
  BattPwrDischrgLmt_kW/1 -> Check Within Limits/1(up)
  BattPwrChrgLmt_kW/1 -> Check Within Limits/3(lo)
  Check Within Limits/2(y) -> ElecToMechPwr/1
  MotEffi2K_1/1 -> ElecToMechPwr/2
  ElecToMechPwr/1 -> MechPwrToTrq/1
  MotSpdAct_rpm/1 -> Abs/1, MechPwrToTrq/2
  Check Within Limits/1(InLimit) -> Switch/2
  MechPwrToTrq/1 -> Switch/3
  MotTrqReqRateLimit_Nm/1 -> Switch1/1, Switch/1
  Switch/1 -> Switch1/3
  Abs/1 -> Compare To Constant/1
  Compare To Constant/1 -> Switch1/2
  Switch1/1 -> MotTrqReqBattPwrLimit_Nm/1

== system EV_Model/VCU/Subsystem/DCU Limit ==
  MotTrqReqBattPwrLimit_Nm : Inport
  DCUPwrLimit_Nm : Inport  Port=2
  DCUTrqLimit_Nm : Inport  Port=3
  Gain : Gain  Gain=-1
  Min : MinMax  Inputs=2
  Saturation Dynamic : simulink/Discontinuities/Saturation Dynamic  OutMin=[]  OutMax=[]  OutDataTypeStr=Inherit: Same as second input  OutDataType=fixdt(1, 16)  OutScaling=2^-10  DoSatur=off
  MotTrqFinalCmd_Nm : Outport  VectorParamsAs1DForOutWhenUnconnected=off
  wires:
  MotTrqReqBattPwrLimit_Nm/1 -> Saturation Dynamic/2
  Saturation Dynamic/1 -> MotTrqFinalCmd_Nm/1
  Gain/1 -> Saturation Dynamic/3
  DCUTrqLimit_Nm/1 -> Min/1
  DCUPwrLimit_Nm/1 -> Min/2
  Min/1 -> Gain/1, Saturation Dynamic/1

== system EV_Model/VCU/Subsystem/Mot Torque Request Cal ==
  note: 轮端到电机扭矩换算
  WhlTrqCmd_Nm : Inport
  VehVelAct_kph : Inport  Port=2
  BattSOC_1 : Inport  Port=3
  DCUTrqLimit_Nm : Inport  Port=4
  Accel Decel Switch : Switch
  Constant4 : Constant  Value=DCU1.FdRatio
  Constant5 : Constant  Value=DCU1.FdEff
  Product7 : Product  Inputs=*//
  Series Regen Braking : Subsystem  InitFcn=%[~]=autosharedicon('autolibutils',gcb,0);  VariantControl=Variant
  MotTrqReq_Nm : Outport  VectorParamsAs1DForOutWhenUnconnected=off
  wires:
  Constant5/1 -> Product7/2
  WhlTrqCmd_Nm/1 -> Product7/1
  Constant4/1 -> Product7/3
  Product7/1 -> Accel Decel Switch/2, Accel Decel Switch/1, Series Regen Braking/1(TrqReq_Nm)
  DCUTrqLimit_Nm/1 -> Series Regen Braking/2(DCUTrqLimit_Nm)
  VehVelAct_kph/1 -> Series Regen Braking/3(VehSpd)
  BattSOC_1/1 -> Series Regen Braking/4(BattSoc)
  Series Regen Braking/1(" MotTrqRegenReq_Nm") -> Accel Decel Switch/3
  Accel Decel Switch/1 -> MotTrqReq_Nm/1

== system EV_Model/VCU/Subsystem/Trq Rate Limit ==
  MotTrqReq_Nm : Inport
  MotSpdAct_rpm : Inport  Port=2
  Add1 : Sum
  Add3 : Sum  Inputs=+-
  Saturation Dynamic : simulink/Discontinuities/Saturation Dynamic  OutMin=[]  OutMax=[]  OutDataTypeStr=Inherit: Same as second input  OutDataType=fixdt(1, 16)  OutScaling=2^-10  DoSatur=off
  Unit Delay : UnitDelay  SampleTime=-1  HasFrameUpgradeWarning=on
  VCU建扭速率限制 : Lookup_n-D  BreakpointsForDimension1=VCU.TrqFilter.TrqAct  BreakpointsForDimension2=VCU.TrqFilter.SpdAct  Table=VCU.TrqFilter.Rate  InternalRulePriority=Speed  RndMeth=Simplest  InputSameDT=on
      settings: InputPortMap=u0,u1
  sample time : Gain  Gain=VCU.sampleTime
  MotTrqReqRateLimit_Nm : Outport
  wires:
  Saturation Dynamic/1 -> MotTrqReqRateLimit_Nm/1, Unit Delay/1
  Add1/1 -> Saturation Dynamic/1
  Add3/1 -> Saturation Dynamic/3
  Unit Delay/1 -> Add1/1, Add3/1
  sample time/1 -> Add1/2, Add3/2
  VCU建扭速率限制/1 -> sample time/1
  MotTrqReq_Nm/1 -> Saturation Dynamic/2, VCU建扭速率限制/1
  MotSpdAct_rpm/1 -> VCU建扭速率限制/2

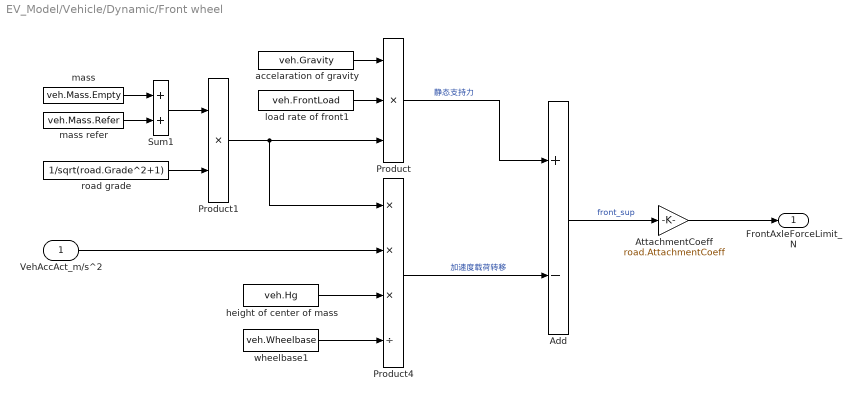
== system EV_Model/Vehicle/Dynamic/Front wheel ==
  VehAccAct_m/s^2 : Inport
  Add : Sum  Inputs=+-
  AttachmentCoeff : Gain  Gain=road.AttachmentCoeff
  Product : Product  Inputs=***
  Product1 : Product  Inputs=**
  Product4 : Product  Inputs=***/
  Sum1 : Sum
  accelaration of gravity : Constant  Value=veh.Gravity
  height of center of mass : Constant  Value=veh.Hg
  load rate of front1 : Constant  Value=veh.FrontLoad
  mass : Constant  Value=veh.Mass.Empty
  mass refer : Constant  Value=veh.Mass.Refer
  road grade : Constant  Value=1/sqrt(road.Grade^2+1)
  wheelbase1 : Constant  Value=veh.Wheelbase
  FrontAxleForceLimit_N : Outport  VectorParamsAs1DForOutWhenUnconnected=off
  wires:
  Product1/1 -> Product4/1, Product/3
  height of center of mass/1 -> Product4/3
  VehAccAct_m/s^2/1 -> Product4/2
  wheelbase1/1 -> Product4/4
  Product4/1 -> Add/2  "加速度载荷转移"
  mass/1 -> Sum1/1
  mass refer/1 -> Sum1/2
  road grade/1 -> Product1/2
  Sum1/1 -> Product1/1
  Product/1 -> Add/1  "静态支持力"
  load rate of front1/1 -> Product/2
  accelaration of gravity/1 -> Product/1
  Add/1 -> AttachmentCoeff/1  "front_sup"
  AttachmentCoeff/1 -> FrontAxleForceLimit_N/1

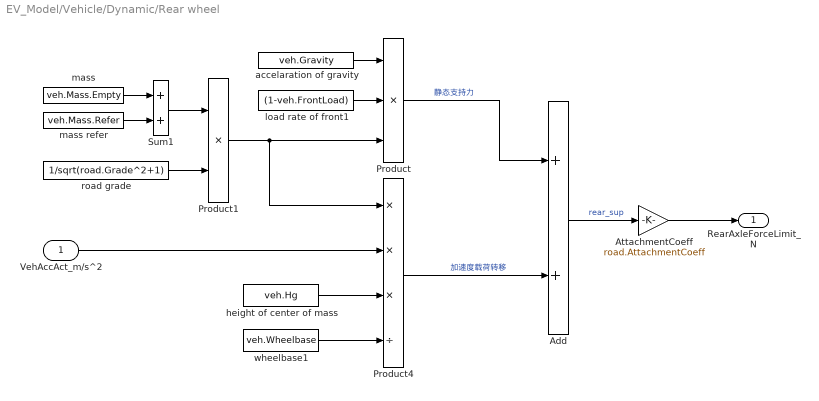
== system EV_Model/Vehicle/Dynamic/Rear wheel ==
  VehAccAct_m/s^2 : Inport
  Add : Sum
  AttachmentCoeff : Gain  Gain=road.AttachmentCoeff
  Product : Product  Inputs=***
  Product1 : Product  Inputs=**
  Product4 : Product  Inputs=***/
  Sum1 : Sum
  accelaration of gravity : Constant  Value=veh.Gravity
  height of center of mass : Constant  Value=veh.Hg
  load rate of front1 : Constant  Value=(1-veh.FrontLoad)
  mass : Constant  Value=veh.Mass.Empty
  mass refer : Constant  Value=veh.Mass.Refer
  road grade : Constant  Value=1/sqrt(road.Grade^2+1)
  wheelbase1 : Constant  Value=veh.Wheelbase
  RearAxleForceLimit_N : Outport  VectorParamsAs1DForOutWhenUnconnected=off
  wires:
  AttachmentCoeff/1 -> RearAxleForceLimit_N/1
  Add/1 -> AttachmentCoeff/1  "rear_sup"
  accelaration of gravity/1 -> Product/1
  load rate of front1/1 -> Product/2
  Product/1 -> Add/1  "静态支持力"
  Sum1/1 -> Product1/1
  road grade/1 -> Product1/2
  mass refer/1 -> Sum1/2
  mass/1 -> Sum1/1
  Product4/1 -> Add/2  "加速度载荷转移"
  wheelbase1/1 -> Product4/4
  VehAccAct_m/s^2/1 -> Product4/2
  height of center of mass/1 -> Product4/3
  Product1/1 -> Product/3, Product4/1

== system EV_Model/Vehicle/Dynamic/Road Ressistance ==
  VehVelAct_kph : Inport
  Compare ToConstant : simulink/Logic and Bit Operations/Compare To Constant  relop=>  const=0  OutDataTypeStr=boolean
  "Fitted Drag Force " : Subsystem
  Grade Resisitance : Subsystem
  Product1 : Product
  Sum2 : Sum
  RoadResis_N : Outport
  wires:
  Grade Resisitance/1(GradeForce_N) -> Sum2/1
  VehVelAct_kph/1 -> Compare ToConstant/1, "Fitted Drag Force "/1(VehVelAct_kph)
  Compare ToConstant/1 -> Product1/1
  Sum2/1 -> Product1/2
  "Fitted Drag Force "/1(WhlForceReq_N) -> Sum2/2
  Product1/1 -> RoadResis_N/1

== system EV_Model/Vehicle/Dynamic/Torque Coordinate ==
  WheelTrqFromMot_Nm : Inport
  WhlTrqCmd_Nm : Inport  Port=2
  Accel Decel Switch : Switch
  Saturation : Saturate  UpperLimit=inf  LowerLimit=0
  Saturation1 : Saturate  UpperLimit=0  LowerLimit=-inf
  Saturation2 : Saturate  UpperLimit=inf  LowerLimit=0
  Subtract : Sum  Inputs=+-
  FricBrakeTrq_Nm : Outport
  WheelTrqAct_Nm : Outport  Port=2
  wires:
  WheelTrqFromMot_Nm/1 -> Accel Decel Switch/2, Saturation/1
  Accel Decel Switch/1 -> WheelTrqAct_Nm/1
  Saturation/1 -> Subtract/1, Accel Decel Switch/3
  WhlTrqCmd_Nm/1 -> Saturation2/1, Saturation1/1
  Saturation1/1 -> Accel Decel Switch/1
  Saturation2/1 -> Subtract/2
  Subtract/1 -> FricBrakeTrq_Nm/1

== system EV_Model/Vehicle/Dynamic/Vehicle Equivalent Mass ==
  Product1 : Product
  Sum2 : Sum
  inertia coefficient : Constant  Value=veh.InerCoeff
  mass_refer : Constant  Value=veh.Mass.Refer
  vehicle mass : Constant  Value=veh.Mass.Empty
  EquivMass_kg : Outport
  wires:
  Product1/1 -> EquivMass_kg/1
  inertia coefficient/1 -> Product1/2
  Sum2/1 -> Product1/1
  vehicle mass/1 -> Sum2/1
  mass_refer/1 -> Sum2/2

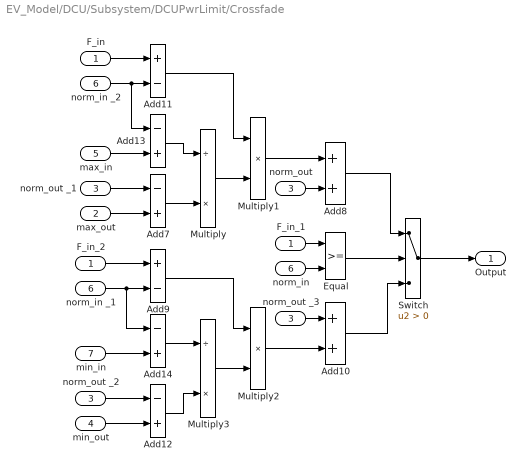
== system EV_Model/DCU/Subsystem/DCUPwrLimit/Crossfade  ==
  F_in : Inport
  max_out : Inport  Port=2
  "norm_out " : Inport  Port=3
  min_out : Inport  Port=4
  max_in : Inport  Port=5
  "norm_in " : Inport  Port=6
  min_in : Inport  Port=7
  Add10 : Sum
  Add11 : Sum  Inputs=+-
  Add{7,12..14} (4 alike) : Sum  Inputs=-+
  Add8 : Sum
  Add9 : Sum  Inputs=+-
  Equal : RelationalOperator  OutDataTypeStr=boolean  RndMeth=Simplest
  F_in_1 : InportShadow
  F_in_2 : InportShadow
  Multiply : Product  Inputs=/*
  Multiply1 : Product  Inputs=**
  Multiply2 : Product  Inputs=**
  Multiply3 : Product  Inputs=/*
  Switch : Switch  Criteria=u2 > Threshold
  norm_in _1 : InportShadow  Port=6
  norm_in _2 : InportShadow  Port=6
  norm_out _1 : InportShadow  Port=3
  norm_out _2 : InportShadow  Port=3
  norm_out _3 : InportShadow  Port=3
  Output : Outport  VectorParamsAs1DForOutWhenUnconnected=off
  wires:
  min_out/1 -> Add12/2
  Add14/1 -> Multiply3/1
  F_in_2/1 -> Add9/1
  Equal/1 -> Switch/2
  F_in_1/1 -> Equal/1
  "norm_in "/1 -> Equal/2
  Multiply2/1 -> Add10/2
  Multiply3/1 -> Multiply2/2
  min_in/1 -> Add14/2
  Multiply/1 -> Multiply1/2
  norm_out _2/1 -> Add12/1
  Add10/1 -> Switch/3
  Add7/1 -> Multiply/2
  Multiply1/1 -> Add8/1
  norm_out _1/1 -> Add7/1
  max_in/1 -> Add13/2
  norm_in _2/1 -> Add11/2, Add13/1
  max_out/1 -> Add7/2
  Add9/1 -> Multiply2/1
  norm_in _1/1 -> Add9/2, Add14/1
  Add13/1 -> Multiply/1
  Switch/1 -> Output/1
  F_in/1 -> Add11/1
  "norm_out "/1 -> Add8/2
  Add12/1 -> Multiply3/2
  norm_out _3/1 -> Add10/1
  Add8/1 -> Switch/1
  Add11/1 -> Multiply1/1

== system EV_Model/DCU/Subsystem/DCUPwrReq/Efficiency ==
  BattVolt_V : Inport
  MotTrqCmd_Nm : Inport  Port=2
  MotSpdAct_rpm : Inport  Port=3
  "Crossfade " : Subsystem  AncestorBlock=GAC_library/Crossfade  mask(Crossfade){}
      mask help: Gradual changing of output in accordance with input siganl F. When the input signal F equals MX, Out equals max. When the input signal F equals NRM, Out equals norm. When the input signal F equals MN, Out equals min. When signal F is between the nominated values of MX/NRM or MN/NRM, then output executes liner interpolation.
      mask Display:
      | color('black')
      | port_label('input', 1, 'F');
      | port_label('input', 2, 'max');
      | port_label('input', 3, 'norm');
      | port_label('input', 4, 'min');
      | port_label('input', 5, 'MX');
      | port_label('input', 6, 'NRM');
      | port_label('input', 7, 'MN');
      | port_label('output',1, 'out');
      | plot(100,100);
      | plot(0,0);
      | color('blue');
      | plot([40 70],[20 20]);
      | plot([40 70],[50 50]);
      | plot([40 70],[80 80]);
      | plot([55 55],[20 80]);
      | text(30,20,'-1');
      | text(30,50,'0');
      | text(30,80,'1');
  DCU1.EffMap(highVolt) : Lookup_n-D  BreakpointsForDimension1=DCU1.EffMap.map1.TrqTab  BreakpointsForDimension2=DCU1.EffMap.map1.SpdTab  Table=DCU1.EffMap.map1.EffTab  InternalRulePriority=Speed  RndMeth=Simplest  InputSameDT=on
      settings: InputPortMap=u0,u1
  DCU1.EffMap(lowVolt) : Lookup_n-D  BreakpointsForDimension1=DCU1.EffMap.map3.TrqTab  BreakpointsForDimension2=DCU1.EffMap.map3.SpdTab  Table=DCU1.EffMap.map3.EffTab  InternalRulePriority=Speed  RndMeth=Simplest  InputSameDT=on
      settings: InputPortMap=u0,u1
  DCU1.EffMap(mediumVolt) : Lookup_n-D  BreakpointsForDimension1=DCU1.EffMap.map2.TrqTab  BreakpointsForDimension2=DCU1.EffMap.map2.SpdTab  Table=DCU1.EffMap.map2.EffTab  InternalRulePriority=Speed  RndMeth=Simplest  InputSameDT=on
      settings: InputPortMap=u0,u1
  MATLAB Function : MATLAB Function  TreatAsAtomicUnit=on
  Saturation : Saturate  UpperLimit=1  LowerLimit=0.2
  Unit Delay : UnitDelay  SampleTime=-1  HasFrameUpgradeWarning=on
  constant1 : Constant  Value=DCU1.EffMap.map1.Volt
  constant2 : Constant  Value=DCU1.EffMap.map2.Volt
  constant3 : Constant  Value=DCU1.EffMap.map3.Volt
  MotEffi_1 : Outport  VectorParamsAs1DForOutWhenUnconnected=off
  wires:
  constant3/1 -> "Crossfade "/7(min_in)
  constant2/1 -> "Crossfade "/6("norm_in ")
  constant1/1 -> "Crossfade "/5(max_in)
  DCU1.EffMap(lowVolt)/1 -> "Crossfade "/4(min_out)
  DCU1.EffMap(mediumVolt)/1 -> "Crossfade "/3("norm_out ")
  DCU1.EffMap(highVolt)/1 -> "Crossfade "/2(max_out)
  "Crossfade "/1(Output) -> Saturation/1
  BattVolt_V/1 -> "Crossfade "/1(F_in)
  Saturation/1 -> MATLAB Function/1(u1)
  Unit Delay/1 -> MATLAB Function/2(u2)
  MATLAB Function/1(y) -> MotEffi_1/1, Unit Delay/1
  MotTrqCmd_Nm/1 -> DCU1.EffMap(highVolt)/1, DCU1.EffMap(mediumVolt)/1, DCU1.EffMap(lowVolt)/1
  MotSpdAct_rpm/1 -> DCU1.EffMap(highVolt)/2, DCU1.EffMap(mediumVolt)/2, DCU1.EffMap(lowVolt)/2

== system EV_Model/DCU/Subsystem/DCUPwrReq/Power ==
  note: Pelec_req = Pmech_req*Eff^k,
      | k = -1 if Motoring >= 0,
      | k = 1 if Generating < 0
  note: Check if Motoring
      | or Generating
  MotEffi_1 : Inport
  MotSpdAct_rpm : Inport  Port=2
  MotTrqCmd_Nm : Inport  Port=3
  Constant1 : Constant  Value=-1  SampleTime=-1
  Constant2 : Constant  SampleTime=-1
  Math Function : Math  Operator=pow  SignedPower=on  OutputSignalType=real  SaturateOnIntegerOverflow=on
  Product4 : Product
  Switch2 : Switch
  "front " : Product  Inputs=**/
  unit conversion factor : Constant  Value=9549
  MotPwrElecReq_kW : Outport  VectorParamsAs1DForOutWhenUnconnected=off
  MotEffi2K_1 : Outport  Port=2  VectorParamsAs1DForOutWhenUnconnected=off
  wires:
  MotSpdAct_rpm/1 -> "front "/1
  unit conversion factor/1 -> "front "/3
  MotTrqCmd_Nm/1 -> "front "/2
  Constant2/1 -> Switch2/3
  Constant1/1 -> Switch2/1
  "front "/1 -> Product4/1, Switch2/2
  Switch2/1 -> Math Function/2
  MotEffi_1/1 -> Math Function/1
  Math Function/1 -> MotEffi2K_1/1, Product4/2
  Product4/1 -> MotPwrElecReq_kW/1

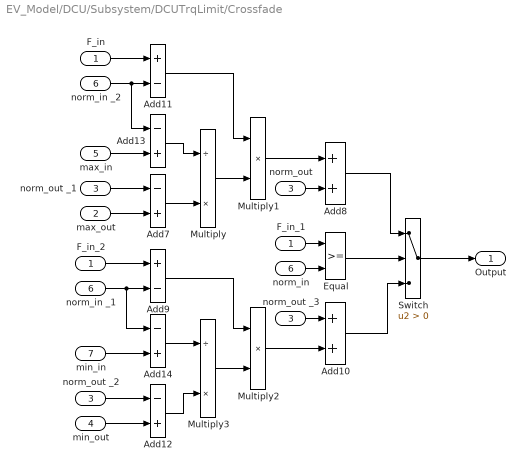
== system EV_Model/DCU/Subsystem/DCUTrqLimit/Crossfade  ==
  F_in : Inport
  max_out : Inport  Port=2
  "norm_out " : Inport  Port=3
  min_out : Inport  Port=4
  max_in : Inport  Port=5
  "norm_in " : Inport  Port=6
  min_in : Inport  Port=7
  Add10 : Sum
  Add11 : Sum  Inputs=+-
  Add{7,12..14} (4 alike) : Sum  Inputs=-+
  Add8 : Sum
  Add9 : Sum  Inputs=+-
  Equal : RelationalOperator  OutDataTypeStr=boolean  RndMeth=Simplest
  F_in_1 : InportShadow
  F_in_2 : InportShadow
  Multiply : Product  Inputs=/*
  Multiply1 : Product  Inputs=**
  Multiply2 : Product  Inputs=**
  Multiply3 : Product  Inputs=/*
  Switch : Switch  Criteria=u2 > Threshold
  norm_in _1 : InportShadow  Port=6
  norm_in _2 : InportShadow  Port=6
  norm_out _1 : InportShadow  Port=3
  norm_out _2 : InportShadow  Port=3
  norm_out _3 : InportShadow  Port=3
  Output : Outport  VectorParamsAs1DForOutWhenUnconnected=off
  wires:
  min_out/1 -> Add12/2
  Add14/1 -> Multiply3/1
  F_in_2/1 -> Add9/1
  Equal/1 -> Switch/2
  F_in_1/1 -> Equal/1
  "norm_in "/1 -> Equal/2
  Multiply2/1 -> Add10/2
  Multiply3/1 -> Multiply2/2
  min_in/1 -> Add14/2
  Multiply/1 -> Multiply1/2
  norm_out _2/1 -> Add12/1
  Add10/1 -> Switch/3
  Add7/1 -> Multiply/2
  Multiply1/1 -> Add8/1
  norm_out _1/1 -> Add7/1
  max_in/1 -> Add13/2
  norm_in _2/1 -> Add11/2, Add13/1
  max_out/1 -> Add7/2
  Add9/1 -> Multiply2/1
  norm_in _1/1 -> Add9/2, Add14/1
  Add13/1 -> Multiply/1
  Switch/1 -> Output/1
  F_in/1 -> Add11/1
  "norm_out "/1 -> Add8/2
  Add12/1 -> Multiply3/2
  norm_out _3/1 -> Add10/1
  Add8/1 -> Switch/1
  Add11/1 -> Multiply1/1

== system EV_Model/Driver/DriverModel/PID/PIDACC ==
  Error : Inport
  reset : Inport  Port=2
  D : Gain  Gain=D  SaturateOnIntegerOverflow=on  OutDataTypeStr=Inherit: Same as input  ParamDataTypeStr=Inherit: Same as input
  Derivative : Derivative
  Discrete-Time Integrator : DiscreteIntegrator  ExternalReset=rising  SampleTime=SampleTime  ICPrevOutput=DiscIntNeverNeededParam  ICPrevScaledInput=DiscIntNeverNeededParam
  Gainintegral1 : Gain  Gain=I  SaturateOnIntegerOverflow=on  OutDataTypeStr=Inherit: Same as input  ParamDataTypeStr=Inherit: Same as input
  Proportional : Gain  Gain=P  SaturateOnIntegerOverflow=on  OutDataTypeStr=Inherit: Same as input  ParamDataTypeStr=Inherit: Same as input
  RateTransition : RateTransition
  Sum : Sum  Inputs=+++  InputSameDT=on  SaturateOnIntegerOverflow=on  OutDataTypeStr=Inherit: Same as first input
  Out_1 : Outport  InitialOutput=0  VectorParamsAs1DForOutWhenUnconnected=off
  wires:
  Sum/1 -> Out_1/1
  D/1 -> RateTransition/1
  Error/1 -> Gainintegral1/1, D/1, Proportional/1
  Derivative/1 -> Sum/3
  Discrete-Time Integrator/1 -> Sum/2
  Gainintegral1/1 -> Discrete-Time Integrator/1
  reset/1 -> Discrete-Time Integrator/2
  RateTransition/1 -> Derivative/1
  Proportional/1 -> Sum/1
